simulink model "JG_shock"  (R2020a)
settings: Solver=VariableStepAuto  StartTime=0.0  StopTime=10.0  RelTol=1e-3
values from neighbouring files (symbols this model uses):
  Gov_spend_to_firms = 0.35    [main.m]
  JG_delay = 1    [main.m]
  JG_salary = 0.3    [main.m]
  Kd = 0.1*10^6    (= 100000)    [main.m]
  Ki = 0.2*10^6    (= 200000)    [main.m]
  Kp = 1*10^6    (= 1000000)    [main.m]
  priv_payroll = 0.5    [main.m]
  Start = 1*10^6    (= 1000000)    [main.m]
  structural_unemp = 0    [main.m]
  target_employment = 2700000    [main.m]
  Tf = 0.3    [main.m]
  Tg = 1    [main.m]
  Tjg = 0.9    [main.m]
  Tpriv = 0.5    [main.m]
  Tpub = 0.5    [main.m]
  Tss = 0.9    [main.m]
  tx_firm = 0.3    [main.m]
  tx_JG = 0.3    [main.m]
  tx_priv = 0.4    [main.m]
  tx_pub = 0.35    [main.m]
  VAT = 0.07    [main.m]
libraries: simulink x1
settings Model: Creator=erlended  LastModifiedBy=erlended

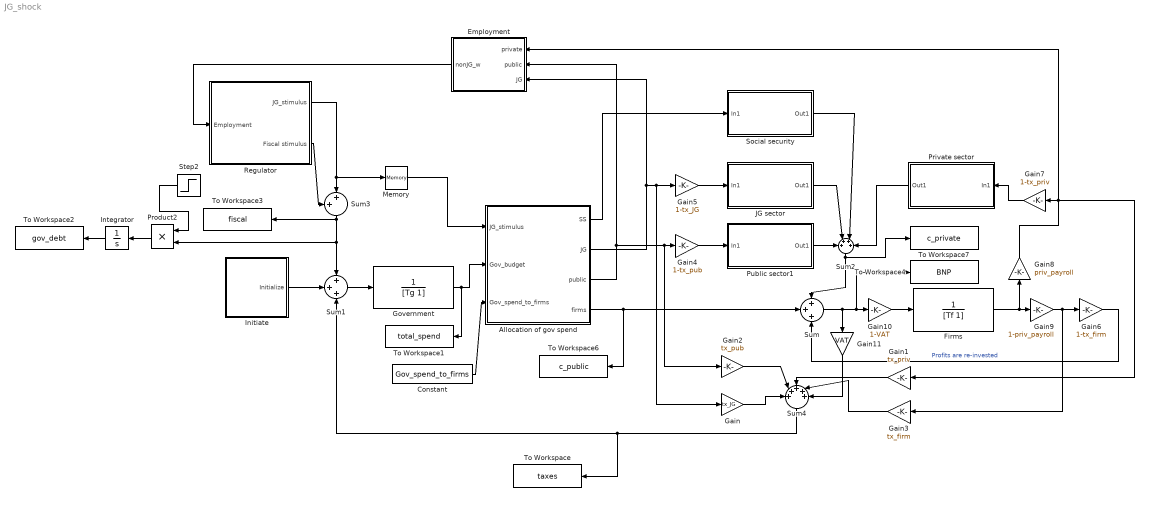
== system JG_shock ==
  Allocation of gov spend : MATLAB Function  TreatAsAtomicUnit=on
  Constant : Constant  Value=Gov_spend_to_firms
  Employment : Subsystem
  Firms : TransferFcn  Denominator=[Tf 1]
  Gain : Gain  Gain=tx_JG
  Gain1 : Gain  Gain=tx_priv
  Gain10 : Gain  Gain=1-VAT
  Gain11 : Gain  Gain=VAT
  Gain2 : Gain  Gain=tx_pub
  Gain3 : Gain  Gain=tx_firm
  Gain4 : Gain  Gain=1-tx_pub
  Gain5 : Gain  Gain=1-tx_JG
  Gain6 : Gain  Gain=1-tx_firm
  Gain7 : Gain  Gain=1-tx_priv
  Gain8 : Gain  Gain=priv_payroll
  Gain9 : Gain  Gain=1-priv_payroll
  Government : TransferFcn  Denominator=[Tg 1]
  Initiate : Subsystem
  Integrator : Integrator
  JG sector : Subsystem
  Memory : Memory
  Private sector : Subsystem
  Product2 : Product
  Public sector1 : Subsystem
  Regulator : Subsystem
  Social security : Subsystem
  Step2 : Step  Time=30  SampleTime=0
  Sum : Sum  Inputs=+++
  Sum1 : Sum  Inputs=+++
  Sum2 : Sum  Inputs=++++
  Sum3 : Sum  Inputs=++|
  Sum4 : Sum  Inputs=+++++
  To Workspace : ToWorkspace  VariableName=taxes  SaveFormat=Timeseries  SampleTime=-1
  To Workspace1 : ToWorkspace  VariableName=total_spend  SaveFormat=Timeseries  SampleTime=-1
  To Workspace2 : ToWorkspace  VariableName=gov_debt  SaveFormat=Timeseries  SampleTime=-1
  To Workspace3 : ToWorkspace  VariableName=fiscal  SaveFormat=Timeseries  SampleTime=-1
  To Workspace4 : ToWorkspace  VariableName=BNP  SaveFormat=Timeseries  SampleTime=-1
  To Workspace6 : ToWorkspace  VariableName=c_public  SaveFormat=Timeseries  SampleTime=-1
  To Workspace7 : ToWorkspace  VariableName=c_private  SaveFormat=Timeseries  SampleTime=-1
  wires:
  Sum1/1 -> Government/1
  Initiate/1(Initialize) -> Sum1/2
  Allocation of gov spend/2(JG) -> Gain5/1, Gain/1, Employment/3(JG)
  Constant/1 -> Allocation of gov spend/3(Gov_spend_to_firms)
  Sum/1 -> Gain11/1, Gain10/1, To Workspace4/1
  Government/1 -> To Workspace1/1, Allocation of gov spend/2(Gov_budget)
  Allocation of gov spend/4(firms) -> To Workspace6/1, Sum/2
  Allocation of gov spend/3(public) -> Employment/2(public), Gain4/1, Gain2/1
  Firms/1 -> Gain8/1, Gain9/1
  Sum2/1 -> Sum/1, To Workspace7/1
  Employment/1(nonJG_w) -> Regulator/1(Employment)
  Regulator/1(JG_stimulus) -> Memory/1, Sum3/2
  Regulator/2(Fiscal stimulus) -> Sum3/1
  Gain/1 -> Sum4/1
  Gain2/1 -> Sum4/2
  Gain1/1 -> Sum4/3
  Gain3/1 -> Sum4/4
  Sum4/1 -> To Workspace/1, Sum1/3
  Gain4/1 -> Public sector1/1(In1)
  Gain5/1 -> JG sector/1(In1)
  Gain7/1 -> Private sector/1(In1)
  Gain9/1 -> Gain6/1, Gain3/1
  Gain8/1 -> Gain1/1, Employment/1(private), Gain7/1
  Gain6/1 -> Sum/3  "Profits are re-invested"
  Public sector1/1(Out1) -> Sum2/1
  JG sector/1(Out1) -> Sum2/2
  Product2/1 -> Integrator/1
  Integrator/1 -> To Workspace2/1
  Step2/1 -> Product2/1
  Sum3/1 -> Sum1/1, Product2/2, To Workspace3/1
  Gain10/1 -> Firms/1
  Gain11/1 -> Sum4/5
  Memory/1 -> Allocation of gov spend/1(JG_stimulus)
  Allocation of gov spend/1(SS) -> Social security/1(In1)
  Private sector/1(Out1) -> Sum2/4
  Social security/1(Out1) -> Sum2/3

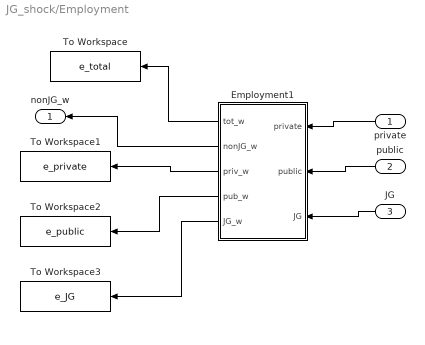
== system JG_shock/Employment ==
  private : Inport
  public : Inport  Port=2
  JG : Inport  Port=3
  Employment1 : MATLAB Function  TreatAsAtomicUnit=on
  To Workspace : ToWorkspace  VariableName=e_total  SaveFormat=Timeseries  SampleTime=-1
  To Workspace1 : ToWorkspace  VariableName=e_private  SaveFormat=Timeseries  SampleTime=-1
  To Workspace2 : ToWorkspace  VariableName=e_public  SaveFormat=Timeseries  SampleTime=-1
  To Workspace3 : ToWorkspace  VariableName=e_JG  SaveFormat=Timeseries  SampleTime=-1
  nonJG_w : Outport
  wires:
  Employment1/1(tot_w) -> To Workspace/1
  Employment1/4(pub_w) -> To Workspace2/1
  Employment1/3(priv_w) -> To Workspace1/1
  public/1 -> Employment1/2(public)
  private/1 -> Employment1/1(private)
  JG/1 -> Employment1/3(JG)
  Employment1/5(JG_w) -> To Workspace3/1
  Employment1/2(nonJG_w) -> nonJG_w/1

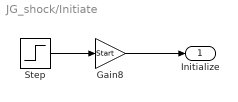
== system JG_shock/Initiate ==
  Gain8 : Gain  Gain=Start
  Step : Step  Before=1  After=0  SampleTime=0
  Initialize : Outport
  wires:
  Step/1 -> Gain8/1
  Gain8/1 -> Initialize/1

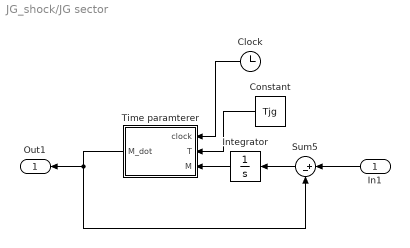
== system JG_shock/JG sector ==
  In1 : Inport
  Clock : Clock
  Constant : Constant  Value=Tjg
  Integrator : Integrator
  Sum5 : Sum  Inputs=|+-
  Time paramterer : MATLAB Function  TreatAsAtomicUnit=on
  Out1 : Outport
  wires:
  Integrator/1 -> Time paramterer/3(M)
  Time paramterer/1(M_dot) -> Out1/1, Sum5/2
  Sum5/1 -> Integrator/1
  In1/1 -> Sum5/1
  Clock/1 -> Time paramterer/1(clock)
  Constant/1 -> Time paramterer/2(T)

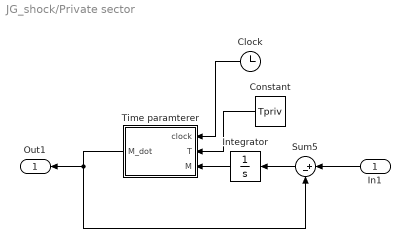
== system JG_shock/Private sector ==
  In1 : Inport
  Clock : Clock
  Constant : Constant  Value=Tpriv
  Integrator : Integrator
  Sum5 : Sum  Inputs=|+-
  Time paramterer : MATLAB Function  TreatAsAtomicUnit=on
  Out1 : Outport
  wires:
  Integrator/1 -> Time paramterer/3(M)
  Time paramterer/1(M_dot) -> Out1/1, Sum5/2
  Sum5/1 -> Integrator/1
  In1/1 -> Sum5/1
  Clock/1 -> Time paramterer/1(clock)
  Constant/1 -> Time paramterer/2(T)

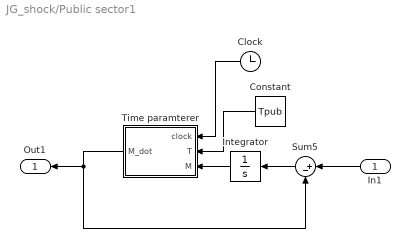
== system JG_shock/Public sector1 ==
  In1 : Inport
  Clock : Clock
  Constant : Constant  Value=Tpub
  Integrator : Integrator
  Sum5 : Sum  Inputs=|+-
  Time paramterer : MATLAB Function  TreatAsAtomicUnit=on
  Out1 : Outport
  wires:
  Integrator/1 -> Time paramterer/3(M)
  Time paramterer/1(M_dot) -> Out1/1, Sum5/2
  Sum5/1 -> Integrator/1
  In1/1 -> Sum5/1
  Clock/1 -> Time paramterer/1(clock)
  Constant/1 -> Time paramterer/2(T)

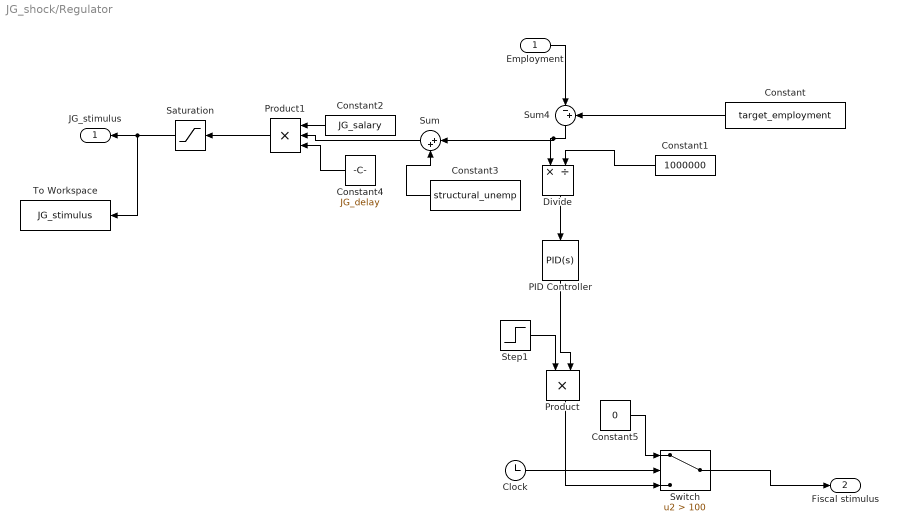
== system JG_shock/Regulator ==
  Employment : Inport
  Clock : Clock
  Constant : Constant  Value=target_employment
  Constant1 : Constant  Value=1000000
  Constant2 : Constant  Value=JG_salary
  Constant3 : Constant  Value=structural_unemp
  Constant4 : Constant  Value=JG_delay
  Constant5 : Constant  Value=0
  Divide : Product  Inputs=*/
  PID Controller : simulink/Continuous/PID Controller  Controller=PID  Form=Parallel  TimeDomain=Continuous-time  UseExternalTs=off  SampleTime=-1  IntegratorMethod=Forward Euler  FilterMethod=Forward Euler  ControllerParametersSource=internal  P=Kp  I=Ki  D=Kd  UseFilter=on  N=1  TunerSelectOption=Transfer Function Based (PID Tuner App)  InitialConditionSource=internal  InitialConditionForIntegrator=0  InitialConditionForFilter=0  DifferentiatorICPrevScaledInput=0  ExternalReset=none  TrackingMode=off  Kt=1  LimitOutput=off  UpperSaturationLimit=inf  LowerSaturationLimit=-inf  LinearizeAsGain=on  AntiWindupMode=none  Kb=1  POutMin=[]  POutMax=[]  IOutMin=[]  IOutMax=[]  DOutMin=[]  DOutMax=[]  NOutMin=[]  NOutMax=[]  SumOutMin=[]  SumOutMax=[]  SaturationOutMin=[]  SaturationOutMax=[]  PParamMin=[]  PParamMax=[]  IParamMin=[]  IParamMax=[]  DParamMin=[]  DParamMax=[]  NParamMin=[]  NParamMax=[]  KbParamMin=[]  KbParamMax=[]  KtParamMin=[]  KtParamMax=[]  KbOutMin=[]  KbOutMax=[]  KtOutMin=[]  KtOutMax=[]  IntegratorOutMin=[]  IntegratorOutMax=[]  FilterOutMin=[]  FilterOutMax=[]  SumI1OutMin=[]  SumI1OutMax=[]  SumI2OutMin=[]  SumI2OutMax=[]  SumI3OutMin=[]  SumI3OutMax=[]  SumI4OutMin=[]  SumI4OutMax=[]  SumDOutMin=[]  SumDOutMax=[]  DifferentiatorOutMin=[]  DifferentiatorOutMax=[]  FilterDiffOutCoefMin=[]  FilterDiffOutCoefMax=[]  ReciprocalOutMin=[]  ReciprocalOutMax=[]  SumDenOutMin=[]  SumDenOutMax=[]  SumNumOutMin=[]  SumNumOutMax=[]  DivideOutMin=[]  DivideOutMax=[]  UdiffTsProdOutMin=[]  UdiffTsProdOutMax=[]  NTsProdOutMin=[]  NTsProdOutMax=[]  UintegralTsProdOutMin=[]  UintegralTsProdOutMax=[]  UngainTsProdOutMin=[]  UngainTsProdOutMax=[]  IntegratorContinuousStateAttributes=''  IntegratorStateMustResolveToSignalObject=off  IntegratorRTWStateStorageClass=Auto  FilterContinuousStateAttributes=''  FilterStateMustResolveToSignalObject=off  FilterRTWStateStorageClass=Auto  ParallelPVariant=InternalParameters  IdealPVariant=Disabled  IVariant=InternalParameters  DVariant=InternalParameters  IntegratorVariant=Continuous  SatVariant=Disabled  AWVariant=Passthrough  PCopyVariant=Disabled  TRVariant=Disabled  FdbkBlocksVariant=Forward  IdealPFdbkVariant=Disabled  SatFdbkVariant=Disabled  DerivativeFilterVariant=ContFilter  NVariant=InternalParameters  NCopyVariant=Disabled  FilterICVariant=InternalICsFilter  IntegratorICVariant=InternalICs  ExternalResetVariant=Disabled  TRSumVariant=Passthrough  SumFdbkVariant=Disabled  SumVariant=Sum_PID  TsampFilterVariant=InternalTs  TsampNgainVariant=Passthrough  TsampIntegralVariant=Passthrough
  Product : Product
  Product1 : Product  Inputs=3
  Saturation : Saturate  UpperLimit=100000000  LowerLimit=0
  Step1 : Step  SampleTime=0
  Sum : Sum  Inputs=|++
  Sum4 : Sum  Inputs=|-+
  Switch : Switch  Criteria=u2 > Threshold  Threshold=100
  To Workspace : ToWorkspace  VariableName=JG_stimulus  SaveFormat=Timeseries  SampleTime=-1
  JG_stimulus : Outport
  Fiscal stimulus : Outport  Port=2
  wires:
  Step1/1 -> Product/1
  PID Controller/1 -> Product/2
  Constant1/1 -> Divide/2
  Divide/1 -> PID Controller/1
  Sum4/1 -> Sum/1, Divide/1
  Employment/1 -> Sum4/1
  Product1/1 -> Saturation/1
  Constant2/1 -> Product1/1
  Saturation/1 -> To Workspace/1, JG_stimulus/1
  Constant/1 -> Sum4/2
  Sum/1 -> Product1/2
  Constant3/1 -> Sum/2
  Constant4/1 -> Product1/3
  Clock/1 -> Switch/2
  Product/1 -> Switch/3
  Constant5/1 -> Switch/1
  Switch/1 -> Fiscal stimulus/1

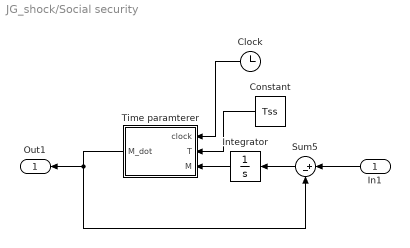
== system JG_shock/Social security ==
  In1 : Inport
  Clock : Clock
  Constant : Constant  Value=Tss
  Integrator : Integrator
  Sum5 : Sum  Inputs=|+-
  Time paramterer : MATLAB Function  TreatAsAtomicUnit=on
  Out1 : Outport
  wires:
  Integrator/1 -> Time paramterer/3(M)
  Time paramterer/1(M_dot) -> Out1/1, Sum5/2
  Sum5/1 -> Integrator/1
  In1/1 -> Sum5/1
  Clock/1 -> Time paramterer/1(clock)
  Constant/1 -> Time paramterer/2(T)

== matlab function JG_shock/Allocation of gov spend ==
  data: SS output; JG output; public output; JG_stimulus input; Gov_budget input; firms output; Gov_spend_to_firms input
function [SS, JG, public, firms] = fcn(JG_stimulus, Gov_budget, Gov_spend_to_firms)
SS = (Gov_budget-JG_stimulus) * 0.3;
public = 0.7*(Gov_budget-JG_stimulus) * (1-Gov_spend_to_firms);
firms = 0.7*(Gov_budget-JG_stimulus) * Gov_spend_to_firms;
JG = JG_stimulus;

== matlab function JG_shock/Employment/Employment1 ==
  data: private input; public input; tot_w output; nonJG_w output; priv_w output; pub_w output; JG input; JG_w output
function  [tot_w, nonJG_w, priv_w, pub_w, JG_w]= fcn(private, public, JG)
private_salary = 0.5; 
public_salary = 0.5;
JG_salary = 0.3;

priv_w = private/private_salary;
pub_w = public/public_salary;
JG_w = JG/JG_salary;

nonJG_w = priv_w + pub_w;
tot_w = priv_w+pub_w+JG_w;

== matlab function JG_shock/Private sector/Time paramterer ==
  data: clock input; T input; M_dot output; M input
function M_dot = fcn(clock, T, M)
temp = 45;
if clock > 30 && clock < 40
    T = T * 1.3;
elseif clock > 40 && clock < 45
    T = T * temp/clock;
end
M_dot = M/T;

== matlab function JG_shock/Public sector1/Time paramterer ==
  data: clock input; T input; M_dot output; M input
function M_dot = fcn(clock, T, M)
temp = 45;
if clock > 30 && clock < 40
    T = T * 1.3;
elseif clock > 40 && clock < 45
    T = T * temp/clock;
end
M_dot = M/T;

== matlab function JG_shock/JG sector/Time paramterer ==
  data: clock input; T input; M_dot output; M input
function M_dot = fcn(clock, T, M)
temp = 45;
if clock > 30 && clock < 40
    T = T * 1.3;
elseif clock > 40 && clock < 45
    T = T * temp/clock;
end
M_dot = M/T;

== matlab function JG_shock/Social security/Time paramterer ==
  data: clock input; T input; M_dot output; M input
function M_dot = fcn(clock, T, M)
temp = 45;
if clock > 30 && clock < 40
    T = T * 1.3;
elseif clock > 40 && clock < 45
    T = T * temp/clock;
end
M_dot = M/T;
